simulink model "PassStCshnFldTrgtPosSelc"  (R2018b)
settings: Solver=FixedStepDiscrete  StartTime=0.0  StopTime=10.0  RelTol=1e-3
undefined symbols (not defined in the file or in its folder): KeSMSwAcsMd30PassStFldUpwdDnwdPos1_Val, KeSMSwAcsMd30PassStFldUpwdDnwdPos1Max_Val, KeSMSwAcsMd30PassStFldUpwdDnwdPos1Min_Val, KeSMSwAcsMd30PassStFldUpwdDnwdPos_Val, KeSMSwAcsMd30PassStFldUpwdDnwdPosMax_Val, KeSMSwAcsMd30PassStFldUpwdDnwdPosMin_Val, KeSMSwAcsMd31PassStFldUpwdDnwdPos_Val, KeSMSwAcsMd31PassStFldUpwdDnwdPosMax_Val, KeSMSwAcsMd31PassStFldUpwdDnwdPosMin_Val, KeSMSwPassStCshnFldEnTrig557BitMask_Val
libraries: TrgtPosSelcLib x3
settings Model: ModifiedHistory=2024.6.26 V3.0.0 557模式流程  Creator=sn2xws  LastModifiedBy=sn2xws
settings DataIOCC: SaveFormat=StructureWithTime
settings OptimizationCC: DefaultParameterBehavior=Inlined  EnhancedBackFolding=on  PassReuseOutputArgsAs=Individual arguments  ZeroExternalMemoryAtStartup=off  ZeroInternalMemoryAtStartup=off  OptimizeBlockOrder=speed  DifferentSizesBufferReuse=on  OptimizationCustomize=off
settings DebuggingCC: ParameterTunabilityLossMsg=error
settings SFSimCC: MATLABDynamicMemAlloc=off
settings RTWCC: SystemTargetFile=autosar.tlc  GenCodeOnly=on  TemplateMakefile=ert_default_tmf  Description=AUTOSAR  GenerateReport=on  IncludeHyperlinkInReport=on  LaunchReport=on  GenerateTraceInfo=on  GenerateTraceReport=on  GenerateTraceReportSl=on  GenerateTraceReportSf=on  GenerateTraceReportEml=on
settings CodeAppCC: ForceParamTrailComments=on  IgnoreCustomStorageClasses=off  OperatorAnnotations=on  SimulinkDataObjDesc=on  SFDataObjDesc=on  InsertBlockDesc=on
settings STFCustomTargetCC: TargetLangStandard=C99 (ISO)  MultiwordLength=256  ParMdlRefBuildCompliant=on  CompOptLevelCompliant=on  IncludeMdlTerminateFcn=off  CombineOutputUpdateFcns=on  SuppressErrorStatus=on  ERTCustomFileBanners=on  SupportNonFinite=off  SupportComplex=off  SupportContinuousTime=off  SupportNonInlinedSFcns=off  RemoveResetFunc=on  MATLABClassNameForMDSCustomization=Simulink.SoftwareTarget.ERTCustomization  AutosarCompliant=on  UseToolchainInfoCompliant=on  LookupTableObjectStructAxisOrder=2,1,3,4,...  LUTObjectStructOrderEvenSpacing=Size,Table,Breakpoints  SystemTargetFile=autosar.tlc
settings ERTTargetCC: TargetLangStandard=C99 (ISO)  ConcurrentExecutionCompliant=off  IncludeMdlTerminateFcn=off  SuppressErrorStatus=on  SupportNonFinite=off  SupportComplex=off  ModelStepFunctionPrototypeControlCompliant=off  CPPClassGenCompliant=off  AutosarCompliant=on  LookupTableObjectStructAxisOrder=2,1,3,4,...  LUTObjectStructOrderEvenSpacing=Size,Table,Breakpoints  InlinedParameterPlacement=NonHierarchical  ERTCustomFileTemplate=example_file_process.tlc  ERTFilePackagingFormat=Compact

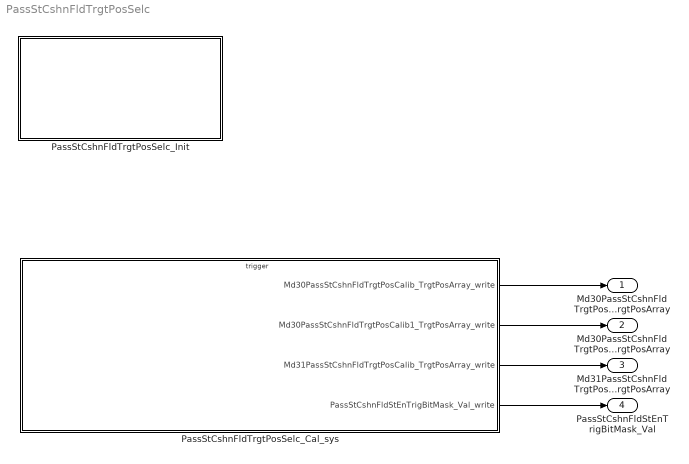
== system PassStCshnFldTrgtPosSelc ==
  PassStCshnFldTrgtPosSelc_Cal_sys : Subsystem
  PassStCshnFldTrgtPosSelc_Init : Subsystem
  Md30PassStCshnFldTrgtPosCalib_TrgtPosArray : Outport  Description=|  OutDataTypeStr=uint16  PortDimensions=3
      | 0:Pos
      | 1:Max
      | 2:Min
  Md30PassStCshnFldTrgtPosCalib1_TrgtPosArray : Outport  Description=|  Port=2  OutDataTypeStr=uint16  PortDimensions=3
      | 0:Pos
      | 1:Max
      | 2:Min
  Md31PassStCshnFldTrgtPosCalib_TrgtPosArray : Outport  Description=|  Port=3  OutDataTypeStr=uint16  PortDimensions=3
      | 0:Pos
      | 1:Max
      | 2:Min
  PassStCshnFldStEnTrigBitMask_Val : Outport  Port=4  OutDataTypeStr=uint32  PortDimensions=1
  wires:
  PassStCshnFldTrgtPosSelc_Cal_sys/1(Md30PassStCshnFldTrgtPosCalib_TrgtPosArray_write) -> Md30PassStCshnFldTrgtPosCalib_TrgtPosArray/1
  PassStCshnFldTrgtPosSelc_Cal_sys/2(Md30PassStCshnFldTrgtPosCalib1_TrgtPosArray_write) -> Md30PassStCshnFldTrgtPosCalib1_TrgtPosArray/1
  PassStCshnFldTrgtPosSelc_Cal_sys/3(Md31PassStCshnFldTrgtPosCalib_TrgtPosArray_write) -> Md31PassStCshnFldTrgtPosCalib_TrgtPosArray/1
  PassStCshnFldTrgtPosSelc_Cal_sys/4(PassStCshnFldStEnTrigBitMask_Val_write) -> PassStCshnFldStEnTrigBitMask_Val/1

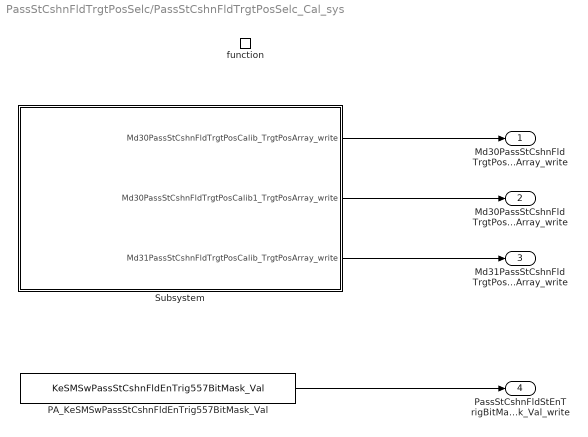
== system PassStCshnFldTrgtPosSelc/PassStCshnFldTrgtPosSelc_Cal_sys ==
  function : TriggerPort  TriggerType=function-call  IsSimulinkFunction=on  FunctionName=PassStCshnFldTrgtPosSelc_Cal  VariantControl=(inherit)
  PA_KeSMSwPassStCshnFldEnTrig557BitMask_Val : Constant  Value=KeSMSwPassStCshnFldEnTrig557BitMask_Val
  Subsystem : Subsystem
  Md30PassStCshnFldTrgtPosCalib_TrgtPosArray_write : Outport
      settings: EnsureOutportIsVirtual=on
  Md30PassStCshnFldTrgtPosCalib1_TrgtPosArray_write : Outport  Port=2
      settings: EnsureOutportIsVirtual=on
  Md31PassStCshnFldTrgtPosCalib_TrgtPosArray_write : Outport  Port=3
      settings: EnsureOutportIsVirtual=on
  PassStCshnFldStEnTrigBitMask_Val_write : Outport  Port=4
      settings: EnsureOutportIsVirtual=on
  wires:
  Subsystem/1(Md30PassStCshnFldTrgtPosCalib_TrgtPosArray_write) -> Md30PassStCshnFldTrgtPosCalib_TrgtPosArray_write/1
  Subsystem/2(Md30PassStCshnFldTrgtPosCalib1_TrgtPosArray_write) -> Md30PassStCshnFldTrgtPosCalib1_TrgtPosArray_write/1
  Subsystem/3(Md31PassStCshnFldTrgtPosCalib_TrgtPosArray_write) -> Md31PassStCshnFldTrgtPosCalib_TrgtPosArray_write/1
  PA_KeSMSwPassStCshnFldEnTrig557BitMask_Val/1 -> PassStCshnFldStEnTrigBitMask_Val_write/1

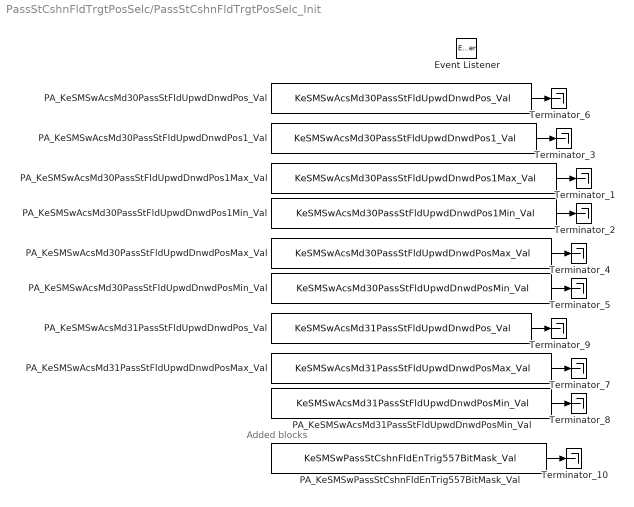
== system PassStCshnFldTrgtPosSelc/PassStCshnFldTrgtPosSelc_Init ==
  note: Added blocks
  Event Listener : EventListener  EventName=reset
  PA_KeSMSwAcsMd30PassStFldUpwdDnwdPos1Max_Val : Constant  Value=KeSMSwAcsMd30PassStFldUpwdDnwdPos1Max_Val
  PA_KeSMSwAcsMd30PassStFldUpwdDnwdPos1Min_Val : Constant  Value=KeSMSwAcsMd30PassStFldUpwdDnwdPos1Min_Val
  PA_KeSMSwAcsMd30PassStFldUpwdDnwdPos1_Val : Constant  Value=KeSMSwAcsMd30PassStFldUpwdDnwdPos1_Val
  PA_KeSMSwAcsMd30PassStFldUpwdDnwdPosMax_Val : Constant  Value=KeSMSwAcsMd30PassStFldUpwdDnwdPosMax_Val
  PA_KeSMSwAcsMd30PassStFldUpwdDnwdPosMin_Val : Constant  Value=KeSMSwAcsMd30PassStFldUpwdDnwdPosMin_Val
  PA_KeSMSwAcsMd30PassStFldUpwdDnwdPos_Val : Constant  Value=KeSMSwAcsMd30PassStFldUpwdDnwdPos_Val
  PA_KeSMSwAcsMd31PassStFldUpwdDnwdPosMax_Val : Constant  Value=KeSMSwAcsMd31PassStFldUpwdDnwdPosMax_Val
  PA_KeSMSwAcsMd31PassStFldUpwdDnwdPosMin_Val : Constant  Value=KeSMSwAcsMd31PassStFldUpwdDnwdPosMin_Val
  PA_KeSMSwAcsMd31PassStFldUpwdDnwdPos_Val : Constant  Value=KeSMSwAcsMd31PassStFldUpwdDnwdPos_Val
  PA_KeSMSwPassStCshnFldEnTrig557BitMask_Val : Constant  Value=KeSMSwPassStCshnFldEnTrig557BitMask_Val
  Terminator_{1..10} (10 alike) : Terminator
  wires:
  PA_KeSMSwAcsMd30PassStFldUpwdDnwdPos1Max_Val/1 -> Terminator_1/1
  PA_KeSMSwAcsMd30PassStFldUpwdDnwdPos1Min_Val/1 -> Terminator_2/1
  PA_KeSMSwAcsMd30PassStFldUpwdDnwdPos1_Val/1 -> Terminator_3/1
  PA_KeSMSwAcsMd30PassStFldUpwdDnwdPosMax_Val/1 -> Terminator_4/1
  PA_KeSMSwAcsMd30PassStFldUpwdDnwdPosMin_Val/1 -> Terminator_5/1
  PA_KeSMSwAcsMd30PassStFldUpwdDnwdPos_Val/1 -> Terminator_6/1
  PA_KeSMSwAcsMd31PassStFldUpwdDnwdPosMax_Val/1 -> Terminator_7/1
  PA_KeSMSwAcsMd31PassStFldUpwdDnwdPosMin_Val/1 -> Terminator_8/1
  PA_KeSMSwAcsMd31PassStFldUpwdDnwdPos_Val/1 -> Terminator_9/1
  PA_KeSMSwPassStCshnFldEnTrig557BitMask_Val/1 -> Terminator_10/1

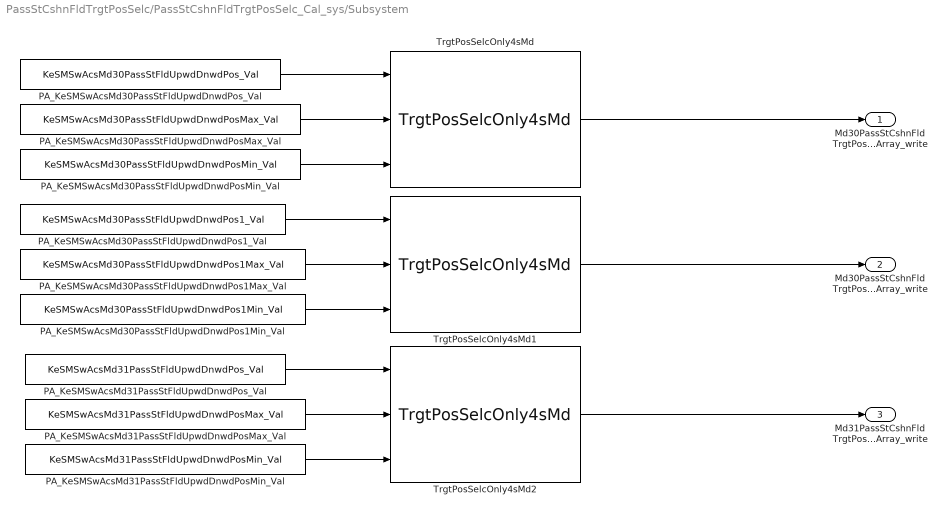
== system PassStCshnFldTrgtPosSelc/PassStCshnFldTrgtPosSelc_Cal_sys/Subsystem ==
  PA_KeSMSwAcsMd30PassStFldUpwdDnwdPos1Max_Val : Constant  Value=KeSMSwAcsMd30PassStFldUpwdDnwdPos1Max_Val
  PA_KeSMSwAcsMd30PassStFldUpwdDnwdPos1Min_Val : Constant  Value=KeSMSwAcsMd30PassStFldUpwdDnwdPos1Min_Val
  PA_KeSMSwAcsMd30PassStFldUpwdDnwdPos1_Val : Constant  Value=KeSMSwAcsMd30PassStFldUpwdDnwdPos1_Val
  PA_KeSMSwAcsMd30PassStFldUpwdDnwdPosMax_Val : Constant  Value=KeSMSwAcsMd30PassStFldUpwdDnwdPosMax_Val
  PA_KeSMSwAcsMd30PassStFldUpwdDnwdPosMin_Val : Constant  Value=KeSMSwAcsMd30PassStFldUpwdDnwdPosMin_Val
  PA_KeSMSwAcsMd30PassStFldUpwdDnwdPos_Val : Constant  Value=KeSMSwAcsMd30PassStFldUpwdDnwdPos_Val
  PA_KeSMSwAcsMd31PassStFldUpwdDnwdPosMax_Val : Constant  Value=KeSMSwAcsMd31PassStFldUpwdDnwdPosMax_Val
  PA_KeSMSwAcsMd31PassStFldUpwdDnwdPosMin_Val : Constant  Value=KeSMSwAcsMd31PassStFldUpwdDnwdPosMin_Val
  PA_KeSMSwAcsMd31PassStFldUpwdDnwdPos_Val : Constant  Value=KeSMSwAcsMd31PassStFldUpwdDnwdPos_Val
  TrgtPosSelcOnly4sMd : TrgtPosSelcLib/TrgtPosSelcOnly4sMd  SystemSampleTime=-1
  TrgtPosSelcOnly4sMd1 : TrgtPosSelcLib/TrgtPosSelcOnly4sMd  SystemSampleTime=-1
  TrgtPosSelcOnly4sMd2 : TrgtPosSelcLib/TrgtPosSelcOnly4sMd  SystemSampleTime=-1
  Md30PassStCshnFldTrgtPosCalib_TrgtPosArray_write : Outport
      settings: EnsureOutportIsVirtual=on
  Md30PassStCshnFldTrgtPosCalib1_TrgtPosArray_write : Outport  Port=2
      settings: EnsureOutportIsVirtual=on
  Md31PassStCshnFldTrgtPosCalib_TrgtPosArray_write : Outport  Port=3
      settings: EnsureOutportIsVirtual=on
  wires:
  TrgtPosSelcOnly4sMd/1 -> Md30PassStCshnFldTrgtPosCalib_TrgtPosArray_write/1
  TrgtPosSelcOnly4sMd1/1 -> Md30PassStCshnFldTrgtPosCalib1_TrgtPosArray_write/1
  TrgtPosSelcOnly4sMd2/1 -> Md31PassStCshnFldTrgtPosCalib_TrgtPosArray_write/1
  PA_KeSMSwAcsMd30PassStFldUpwdDnwdPosMax_Val/1 -> TrgtPosSelcOnly4sMd/2
  PA_KeSMSwAcsMd30PassStFldUpwdDnwdPosMin_Val/1 -> TrgtPosSelcOnly4sMd/3
  PA_KeSMSwAcsMd30PassStFldUpwdDnwdPos_Val/1 -> TrgtPosSelcOnly4sMd/1
  PA_KeSMSwAcsMd30PassStFldUpwdDnwdPos1Max_Val/1 -> TrgtPosSelcOnly4sMd1/2
  PA_KeSMSwAcsMd30PassStFldUpwdDnwdPos1Min_Val/1 -> TrgtPosSelcOnly4sMd1/3
  PA_KeSMSwAcsMd30PassStFldUpwdDnwdPos1_Val/1 -> TrgtPosSelcOnly4sMd1/1
  PA_KeSMSwAcsMd31PassStFldUpwdDnwdPosMax_Val/1 -> TrgtPosSelcOnly4sMd2/2
  PA_KeSMSwAcsMd31PassStFldUpwdDnwdPosMin_Val/1 -> TrgtPosSelcOnly4sMd2/3
  PA_KeSMSwAcsMd31PassStFldUpwdDnwdPos_Val/1 -> TrgtPosSelcOnly4sMd2/1
